simulink model "a9"  (R2016a)
settings: Solver=VariableStepAuto  StartTime=0.0  StopTime=10.0  RelTol=1e-3
settings Model: Creator=user  LastModifiedBy=user

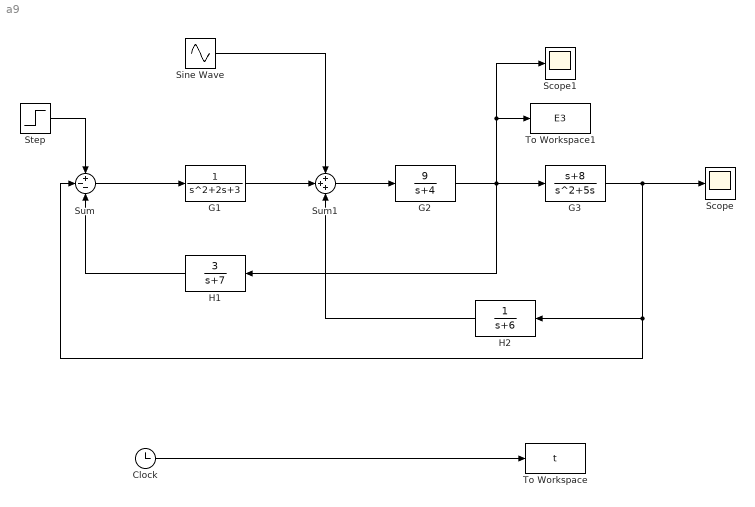
== system a9 ==
  Clock : Clock
  G1 : TransferFcn  Denominator=[1 2 3]
  G2 : TransferFcn  Numerator=[9]  Denominator=[1 4]
  G3 : TransferFcn  Numerator=[1 8]  Denominator=[1 5 0]
  H1 : TransferFcn  Numerator=[3]  Denominator=[1 7]
  H2 : TransferFcn  Denominator=[1 6]
  Scope : Scope
  Scope1 : Scope
  Sine Wave : Sin  Amplitude=0.2  Frequency=2  SampleTime=0
  Step : Step  Time=0  SampleTime=0
  Sum : Sum  Inputs=+--
  Sum1 : Sum  Inputs=+++
  To Workspace : ToWorkspace  VariableName=t  SampleTime=-1
  To Workspace1 : ToWorkspace  VariableName=E3  SampleTime=-1
  wires:
  Sum/1 -> G1/1
  G1/1 -> Sum1/2
  Sine Wave/1 -> Sum1/1
  Sum1/1 -> G2/1
  G2/1 -> To Workspace1/1, Scope1/1, H1/1, G3/1
  G3/1 -> Sum/2, H2/1, Scope/1
  H2/1 -> Sum1/3
  H1/1 -> Sum/3
  Step/1 -> Sum/1
  Clock/1 -> To Workspace/1
